simulink model "SOB_PMSM_NNSMC_20241219"  (R2024b)
settings: Solver=FixedStepDiscrete  StartTime=0.0  StopTime=30  FixedStep=1/20000  RelTol=1e-3
values from neighbouring files (symbols this model uses):
  id2_init = [i2]'    [SOB_PMSM_Fullstate_Feedback_Parameter.m]    (also in SOB_PMSM_NNSMC_Parameter.m)
undefined symbols (not defined in the file or in its folder): DiscIntNeverNeededParam
libraries: simulink x3
settings Model: Creator=COLAB  LastModifiedBy=user
settings SolverCC: AlgebraicLoopSolver=TrustRegion
settings RTWCC: GPUComputeCapability=3.5

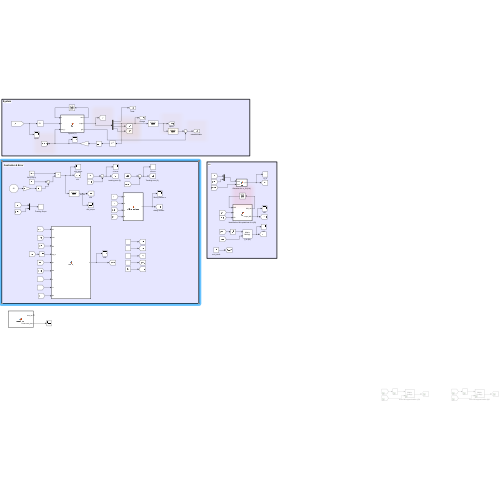
[thumbnail: Simulink's stored preview of the top-level diagram]
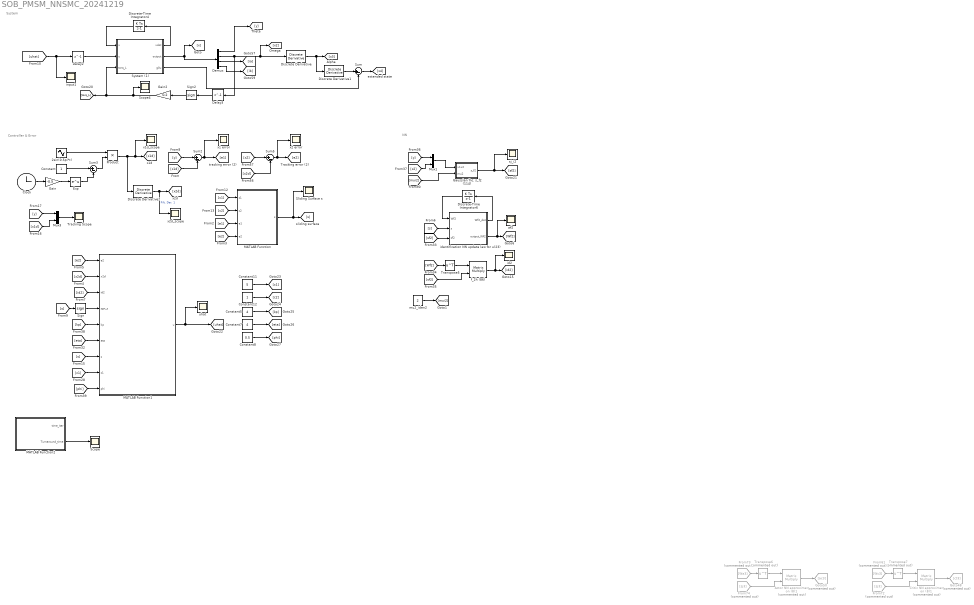
== system SOB_PMSM_NNSMC_20241219 ==
  note: System
  note: Controller & Error
  note: NN
  2sin(0.5pi*t) : Sin  Amplitude=2  Frequency=0.5*pi  SampleTime=0
  Actor NN approximation (8)1 : Product  Commented=on  Multiplication=Matrix(*)
  Clock : Clock
  Constant : Constant
  Constant11 : Constant  Value=5
  Constant12 : Constant
  Constant5 : Constant  Value=4
  Constant7 : Constant  Value=4
  Constant8 : Constant  Value=0.5
  Critic NN approximation (8)1 : Product  Commented=on  Multiplication=Matrix(*)
  Delay2 : Delay  DelayLength=1
  Delay3 : Delay  DelayLength=1
  Demux : Demux
  Discrete Derivative : simulink/Discrete/Discrete Derivative  gainval=1.0  ICPrevScaledInput=0.0  OutMin=[]  OutMax=[]  OutDataType=fixdt(1, 16)  OutScaling=2^-10  DoSatur=off
  Discrete Derivative1 : simulink/Discrete/Discrete Derivative  gainval=1.0  ICPrevScaledInput=0.0  OutMin=[]  OutMax=[]  OutDataType=fixdt(1, 16)  OutScaling=2^-10  DoSatur=off
  Discrete Derivative2 : simulink/Discrete/Discrete Derivative  gainval=1.0  ICPrevScaledInput=0.0  OutMin=[]  OutMax=[]  OutDataType=fixdt(1, 16)  OutScaling=2^-10  DoSatur=off
  Discrete-Time Integrator4 : DiscreteIntegrator  InitialCondition=[0 0 0 0]  SampleTime=-1  ICPrevOutput=DiscIntNeverNeededParam  ICPrevScaledInput=DiscIntNeverNeededParam
  Discrete-Time Integrator6 : DiscreteIntegrator  InitialCondition=id2_init  SampleTime=-1  ICPrevOutput=DiscIntNeverNeededParam  ICPrevScaledInput=DiscIntNeverNeededParam
  Exp : Math
  From61 : From  Commented=on  GotoTag=Wc3
  From72 : From  Commented=on  GotoTag=sj3
  From73 : From  Commented=on  GotoTag=Wa3
  From74 : From  Commented=on  GotoTag=sj3
  Gain : Gain  Gain=-0.5
  Gain2 : Gain  Gain=0.2
  Gaussian fnc. s_f2 (114) : MATLAB Function  TreatAsAtomicUnit=on
  Goto48 : Goto  Commented=on  GotoTag=ct3
  Goto50 : Goto  Commented=on  GotoTag=ac3
  MATLAB Function : MATLAB Function  TreatAsAtomicUnit=on
  MATLAB Function1 : MATLAB Function  TreatAsAtomicUnit=on
  MATLAB Function2 : MATLAB Function  TreatAsAtomicUnit=on
  Mux1 : Mux  Inputs=2
  Mux3 : Mux  Inputs=2
  Product : Product
  Scope : Scope
  Scope4 : Scope
  Sign : Signum
  Sign2 : Signum
  Sliding Surface s : Scope
  Sum{,2..3,5} (4 alike) : Sum  Inputs=|+-
  System (1) : MATLAB Function  TreatAsAtomicUnit=on
  Tracking Scope : Scope
  Transpose5 : Math  Operator=transpose  SignedPower=on
  Transpose6 : Math  Commented=on  Operator=transpose  SignedPower=on
  Transpose7 : Math  Commented=on  Operator=transpose  SignedPower=on
  f_2h (86) : Product  Multiplication=Matrix(*)
  id2 : Scope
  identification NN update law for u(23) : MATLAB Function  TreatAsAtomicUnit=on
  input1 : Scope
  mu2_iden2 : Constant  Value=2
  sj_i2 : Scope
  uhat : Scope
  wf2 : Scope
  x1 error : Scope
  x1d_scope : Scope
  x2 error : Scope
  x2d_scope : Scope
  wires:
  Gain/1 -> Exp/1
  Sum3/1 -> Product/2
  Product/1 -> Discrete Derivative2/1, x1d_scope/1, [x1d]
  Exp/1 -> Sum3/2
  Constant/1 -> Sum3/1
  Clock/1 -> Gain/1
  Mux3/1 -> Tracking Scope/1
  [x1d] -> Mux3/2
  [y] -> Mux3/1
  Sum2/1 -> [e1], x1 error/1
  [y] -> Sum2/1
  [x1d] -> Sum2/2
  2sin(0.5pi*t)/1 -> Product/1
  Sum5/1 -> [e2], x2 error/1
  [x2] -> Sum5/1
  [x2d] -> Sum5/2
  Gaussian fnc. s_f2 (114)/1(s_f2) -> [sf2], sj_i2/1
  [x2] -> Mux1/2
  Mux1/1 -> Gaussian fnc. s_f2 (114)/1(x1x2)
  [y] -> Mux1/1
  identification NN update law for u(23)/1(Wf2_dot) -> Discrete-Time Integrator6/1
  Discrete-Time Integrator6/1 -> identification NN update law for u(23)/1(Wf2)
  [sf2] -> identification NN update law for u(23)/3(sf2)
  identification NN update law for u(23)/2(output_Wf2) -> [Wf2], wf2/1
  [Wf2] -> Transpose5/1
  Transpose5/1 -> f_2h (86)/1
  [sf2] -> f_2h (86)/2
  f_2h (86)/1 -> id2/1, [id2]
  Critic NN approximation (8)1/1 -> Goto48/1
  From72/1 -> Critic NN approximation (8)1/2
  Transpose7/1 -> Critic NN approximation (8)1/1
  From61/1 -> Transpose7/1
  From73/1 -> Transpose6/1
  Transpose6/1 -> Actor NN approximation (8)1/1
  From74/1 -> Actor NN approximation (8)1/2
  Actor NN approximation (8)1/1 -> Goto50/1
  Demux/4 -> [ib]
  Demux/3 -> [ia]
  [uhat] -> Delay2/1, input1/1
  Discrete-Time Integrator4/1 -> System (1)/1(x)
  System (1)/1(xdot) -> Discrete-Time Integrator4/1
  Demux/2 -> Delay3/1, Discrete Derivative/1, [x2]
  Demux/1 -> [y]
  Sign2/1 -> Gain2/1
  Discrete Derivative/1 -> Discrete Derivative1/1, [x3]
  Gain2/1 -> System (1)/3(torq_L), [torq_L], Scope4/1
  System (1)/2(output) -> Demux/1, [x]
  Discrete Derivative1/1 -> Sum/1
  System (1)/3(g0u) -> Sum/2
  Sum/1 -> [x4]
  [mui2] -> Gaussian fnc. s_f2 (114)/2(mu2)
  Delay2/1 -> System (1)/2(u)
  Delay3/1 -> Sign2/1
  Discrete Derivative2/1 -> x2d_scope/1, [x2d]  "Filt. Der. 1"
  [e1] -> MATLAB Function/3(e1)
  [e2] -> MATLAB Function/4(e2)
  [c1] -> MATLAB Function/1(c1)
  [c2] -> MATLAB Function/2(c2)
  [s] -> Sign/1
  [e2] -> MATLAB Function1/1(e2)
  [x2d] -> MATLAB Function1/2(x2d)
  [id2] -> MATLAB Function1/3(id2)
  [s] -> MATLAB Function1/7(s)
  Sign/1 -> MATLAB Function1/4(sgn_s)
  [kp] -> MATLAB Function1/5(kp)
  [eta] -> MATLAB Function1/6(eta)
  MATLAB Function1/1(u) -> uhat/1, [uhat]
  mu2_iden2/1 -> [mui2]
  [s] -> identification NN update law for u(23)/2(s)
  MATLAB Function/1(s) -> Sliding Surface s/1, [s]
  [c1] -> MATLAB Function1/8(c1)
  Constant11/1 -> [c1]
  Constant12/1 -> [c2]
  Constant7/1 -> [eta]
  Constant5/1 -> [kp]
  Constant8/1 -> [phi]
  [phi] -> MATLAB Function1/9(phi)
  MATLAB Function2/2(Turnaround_time) -> Scope/1

== matlab function SOB_PMSM_NNSMC_20241219/Gaussian fnc. s_f2 (114) ==
  data: x1x2 input size=2; s_f2 output size=16; mean3 parameter; mu2 input
function s_f2 = fcn(x1x2,mean3, mu2)

s_fm2 = [0 0 0 0 0 0 0 0 0 0 0 0 0 0 0 0];

for i=1:16
    s_fm2(i)=gau(i);
end

s_f2 = [s_fm2]';

function y = gau(x)
    y = exp(-(norm(x1x2+mean3(x,:)'))^(2)/(mu2^(2)));
end

end

== matlab function SOB_PMSM_NNSMC_20241219/System (1) ==
  data: x input; u input; xdot output; torq_L input; output output; g0u output
function [xdot, output, g0u] = fcn(x, u, torq_L)

Psi       = 0.017;
PolePairs = 4.0;

Km=1.5*Psi*PolePairs;
L=0.4e-3;
J=4.675e-4;
R=0.2;
P=4;
B=2.1e-3;
g0=0.01;

va=-u*sin(P*x(1));
vb=u*cos(P*x(1));
Omega_dot=(1/J)*(-Km*x(3)*sin(P*x(1))+Km*x(4)*cos(P*x(1))-B*x(2)-torq_L);
ia_dot=(1/L)*(va-R*x(3)+Km*x(2)*sin(P*x(1)));
ib_dot=(1/L)*(vb-R*x(4)-Km*x(2)*cos(P*x(1)));

xdot=[x(2) Omega_dot ia_dot ib_dot];

g0u=(g0*Km/(J*L))*u;
output=x;

== matlab function SOB_PMSM_NNSMC_20241219/MATLAB Function ==
  data: c1 input; s output; c2 input; e1 input; e2 input
function s = sliding_surface(c1, c2, e1, e2)

s = c1*e1 + c2*e2;

== matlab function SOB_PMSM_NNSMC_20241219/MATLAB Function2 ==
  data: time_iter output; Turnaround_time output
function [time_iter, Turnaround_time] = toggle_flag()
% time_iter: 0 또는 1로 반복적으로 변하는 출력 변수
% Turnaround_time: 측정된 작업 시간

% Persistent 변수 선언
persistent counter;
persistent stored_Turnaround_time;

% Persistent 변수 초기화
if isempty(counter)
    counter = 0; % 초기 상태 설정
end

if isempty(stored_Turnaround_time)
    stored_Turnaround_time = 0; % 초기 상태 설정
end

% 현재 상태 반환
time_iter = mod(counter, 2); % 0 또는 1을 반환

% Task Turnaround Time 측정
if time_iter == 0
    tic;
    Turnaround_time = stored_Turnaround_time; % 이전 측정값 반환
else
    stored_Turnaround_time = toc;
    Turnaround_time = stored_Turnaround_time; % 현재 측정값 반환
    fprintf('Fullstate Feedback Case Turn around time : %.12f\n', Turnaround_time);
end

% counter 증가
counter = counter + 1;

end

== matlab function SOB_PMSM_NNSMC_20241219/MATLAB Function1 ==
  data: e2 input; u output; x2d input; id2 input; sgn_s input; kp input; eta input; s input; c1 input; phi input
function u = NNSMC(e2, x2d, id2, sgn_s, kp, eta, s, c1, phi)

u_eq = -c1*e2 + x2d - id2;
if abs(s) >= phi
    u_sw = -kp*s -eta*sgn_s;
else
    u_sw = -kp*s;
end

u = u_eq+u_sw;

== matlab function SOB_PMSM_NNSMC_20241219/identification NN update law for u(23) ==
  data: Wf2 input; s input; Wf2_dot output; output_Wf2 output; sf2 input
function [Wf2_dot, output_Wf2] = fcn(Wf2, s, sf2)

GAMMA2=diag([1 1 1 1 1 1 1 1 1 1 1 1 1 1 1 1]).*(0.5);
sigma2=15.8;

Wf2_dot = [GAMMA2*(sf2*s-sigma2*Wf2)];

output_Wf2=Wf2;
